simulink model "Approximation"  (R2024a)
settings: Solver=VariableStepAuto  StartTime=0.0  StopTime=15  RelTol=1e-3
values from neighbouring files (symbols this model uses):
  K = K(:,:,VeloIndexK)    [loadSystem.m]
  relOutput = 1:1:length(K.InputName)    [loadSystem.m]
  sysOL = sysOL(relOutput,:,VeloIndexSys)    [loadSystem.m]
settings Model: Creator=sp-ma  LastModifiedBy=sp-ma

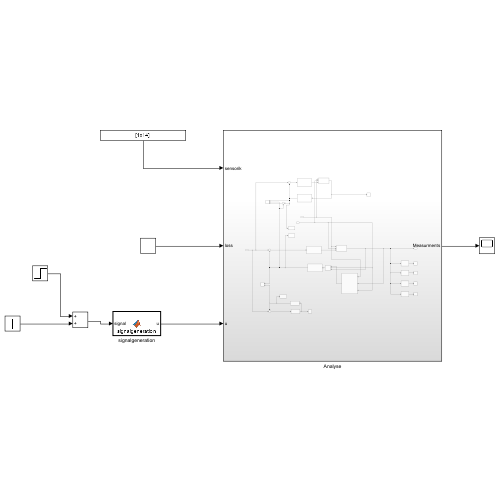
[thumbnail: Simulink's stored preview of the top-level diagram]
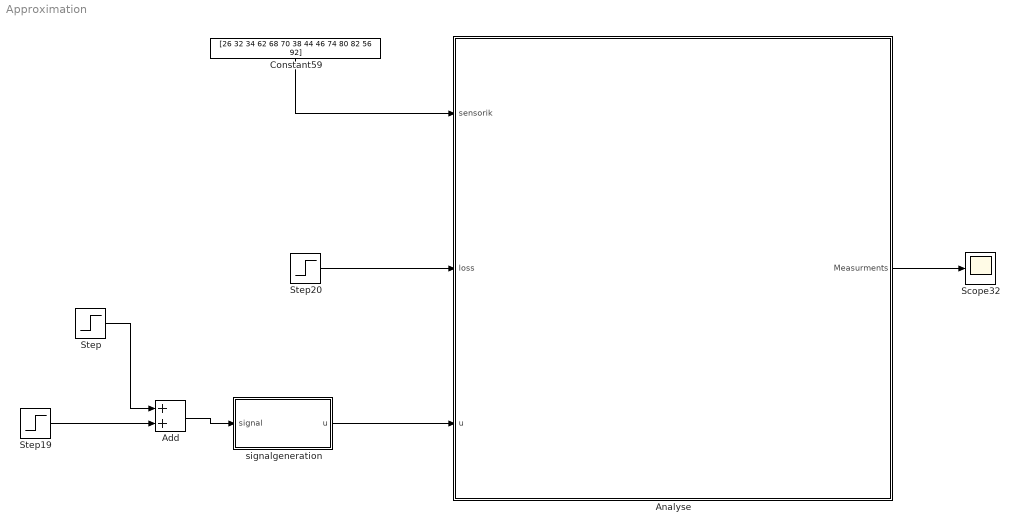
== system Approximation ==
  Add : Sum
  Analyse : Subsystem
  Constant59 : Constant  Value=[26 32 34 62 68 70 38 44 46 74 80 82 56 92]  VectorParams1D=off
  Scope32 : Scope
  Step : Step  Time=0.5  After=0  SampleTime=0
  Step19 : Step  Before=0.1  After=0.1  SampleTime=0
  Step20 : Step  Time=0.5  Before=1  SampleTime=0
  signalgeneration : MATLAB Function  TreatAsAtomicUnit=on
  wires:
  Constant59/1 -> Analyse/1(sensorik)
  Step20/1 -> Analyse/2(loss)
  signalgeneration/1(u) -> Analyse/3(u)
  Analyse/1(Measurments) -> Scope32/1
  Step19/1 -> Add/2
  Step/1 -> Add/1
  Add/1 -> signalgeneration/1(signal)

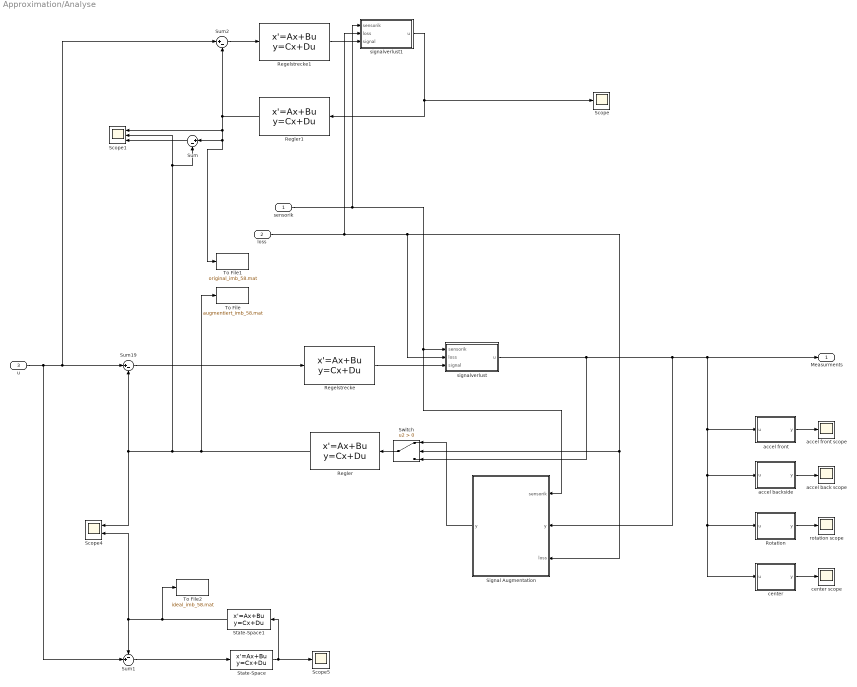
== system Approximation/Analyse ==
  sensorik : Inport
  loss : Inport  Port=2
  u : Inport  Port=3
  Regelstrecke : StateSpace  A=sysOL.A  B=sysOL.B  C=sysOL.C  D=sysOL.D  InitialCondition=0
  Regelstrecke1 : StateSpace  A=sysOL.A  B=sysOL.B  C=sysOL.C  D=sysOL.D  InitialCondition=0
  Regler : StateSpace  A=K.A  B=K.B  C=K.C  D=K.D  InitialCondition=0
  Regler1 : StateSpace  A=K.A  B=K.B  C=K.C  D=K.D  InitialCondition=0
  Rotation : MATLAB Function  TreatAsAtomicUnit=on
  Scope : Scope
  Scope1 : Scope  NumInputPorts=3
  Scope4 : Scope  NumInputPorts=2
  Scope5 : Scope
  Signal Augmentation : Subsystem
  State-Space : StateSpace  A=sysOL.A  B=sysOL.B  C=sysOL.C(relOutput,:)  D=sysOL.D(relOutput,:)  InitialCondition=0
  State-Space1 : StateSpace  A=K.A  B=K.B  C=K.C  D=K.D  InitialCondition=0
  Sum : Sum  Inputs=|+-
  Sum1 : Sum  Inputs=-+|
  Sum19 : Sum  Inputs=|+-
  Sum2 : Sum  Inputs=|+-
  Switch : Switch  Criteria=u2 > Threshold  SaturateOnIntegerOverflow=off  InputSameDT=off
  To File : ToFile  Filename=augmentiert_imb_58.mat
  To File1 : ToFile  Filename=original_imb_58.mat
  To File2 : ToFile  Filename=ideal_imb_58.mat
  accel back scope : Scope
  accel backside : MATLAB Function  TreatAsAtomicUnit=on
  accel front : MATLAB Function  TreatAsAtomicUnit=on
  accel front scope : Scope
  center : MATLAB Function  TreatAsAtomicUnit=on
  center scope : Scope
  rotation scope : Scope
  signalverlust : MATLAB Function  TreatAsAtomicUnit=on
  signalverlust1 : MATLAB Function  TreatAsAtomicUnit=on
  Measurments : Outport
  wires:
  sensorik/1 -> signalverlust1/1(sensorik), signalverlust/1(sensorik), Signal Augmentation/1(sensorik)
  u/1 -> Sum1/2, Sum2/1, Sum19/1
  Regelstrecke/1 -> signalverlust/3(signal)
  Regler/1 -> To File/1, Sum/2, Scope1/2, Sum19/2, Scope4/1
  Switch/1 -> Regler/1
  Rotation/1(y) -> rotation scope/1
  accel backside/1(y) -> accel back scope/1
  accel front/1(y) -> accel front scope/1
  signalverlust/1(u) -> accel front/1(u), accel backside/1(u), center/1(u), Rotation/1(u), Measurments/1, Signal Augmentation/2("y "), Switch/3
  loss/1 -> signalverlust1/2(loss), Signal Augmentation/3(loss), Switch/2, signalverlust/2(loss)
  Signal Augmentation/1(y) -> Switch/1
  State-Space1/1 -> To File2/1, Sum1/1, Scope4/2
  Sum1/1 -> State-Space/1
  State-Space/1 -> Scope5/1, State-Space1/1
  center/1(y) -> center scope/1
  Sum19/1 -> Regelstrecke/1
  Regelstrecke1/1 -> signalverlust1/3(signal)
  signalverlust1/1(u) -> Scope/1, Regler1/1
  Sum2/1 -> Regelstrecke1/1
  Regler1/1 -> To File1/1, Sum/1, Scope1/1, Sum2/2
  Sum/1 -> Scope1/3

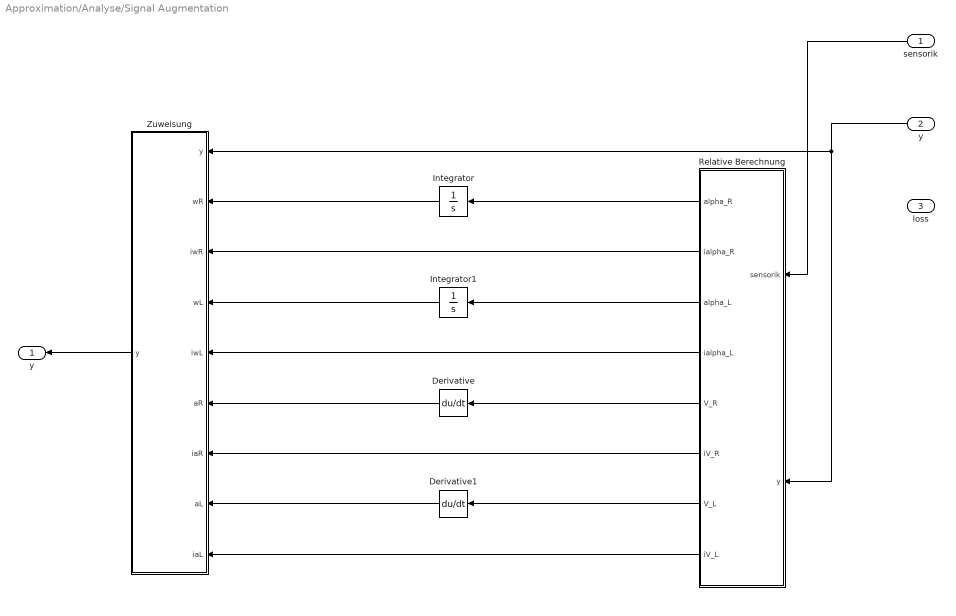
== system Approximation/Analyse/Signal Augmentation ==
  sensorik : Inport
  "y " : Inport  Port=2
  loss : Inport  Port=3
  Derivative : Derivative
  Derivative1 : Derivative
  Integrator : Integrator
  Integrator1 : Integrator
  Relative Berechnung : MATLAB Function  TreatAsAtomicUnit=on
  Zuweisung : MATLAB Function  TreatAsAtomicUnit=on
  y : Outport
  wires:
  Relative Berechnung/5(V_R) -> Derivative/1
  Relative Berechnung/6(iV_R) -> Zuweisung/7(iaR)
  Relative Berechnung/1(alpha_R) -> Integrator/1
  sensorik/1 -> Relative Berechnung/1(sensorik)
  Zuweisung/1(y) -> y/1
  Relative Berechnung/2(ialpha_R) -> Zuweisung/3(iwR)
  Relative Berechnung/8(iV_L) -> Zuweisung/9(iaL)
  Derivative1/1 -> Zuweisung/8(aL)
  Integrator/1 -> Zuweisung/2(wR)
  Relative Berechnung/4(ialpha_L) -> Zuweisung/5(iwL)
  Relative Berechnung/3(alpha_L) -> Integrator1/1
  Relative Berechnung/7(V_L) -> Derivative1/1
  "y "/1 -> Relative Berechnung/2(y), Zuweisung/1("y ")
  Derivative/1 -> Zuweisung/6(aR)
  Integrator1/1 -> Zuweisung/4(wL)

== matlab function Approximation/Analyse/center ==
  data: u input; y output
function y = fcn(u)
rot = [7 12];
y = u(rot);

== matlab function Approximation/Analyse/signalverlust1 ==
  data: sensorik input; loss input; u output; signal input
function u = signalverlust(sensorik,loss,signal)

if(loss~=0)
    signal(sensorik)=0;
end
u=signal;

== matlab function Approximation/signalgeneration ==
  data: u output; signal input
function u = signalgeneration(signal)
% t =0:10;
command = zeros(19,1);
% ilaileron = 13;
% iraileron = 14;
% command([15:19])=sin(t);
% % command([iraileron])=-1;

command([15 16]) = signal;
command([17 18]) = signal;
u=command;

== matlab function Approximation/Analyse/signalverlust ==
  data: sensorik input; loss input; u output; signal input
function u = signalverlust(sensorik,loss,signal)

if(loss~=0)
    signal(sensorik)=0;
end
u=signal;

== matlab function Approximation/Analyse/accel front ==
  data: u input; y output
function y = fcn(u)
fw = [26 38 50 62 74 86];
y = u(fw);

== matlab function Approximation/Analyse/accel backside ==
  data: u input; y output
function y = fcn(u)
bw = [32 44 56 68 80 92];
y = u(bw);

== matlab function Approximation/Analyse/Rotation ==
  data: u input; y output
function y = fcn(u)
rot = [34 46 58 70 82 94];
y = u(rot);

== matlab function Approximation/Analyse/Signal Augmentation/Relative Berechnung ==
  data: sensorik input; alpha_R output; ialpha_R output; alpha_L output; ialpha_L output; y input; V_R output; iV_R output; V_L output; iV_L output
function [alpha_R,ialpha_R,alpha_L,ialpha_L,V_R,iV_R,V_L,iV_L] = fcn(sensorik,y)

%Indexe der Sensoren der Flügelquerschnitte links und rechts fw=forward;
%bw = backward; rot = rotation
    Rfw =  [62 74 86];
    Rbw =  [68 80 92];
    Rrot = [70 82 94];
    R = [Rfw;Rbw;Rrot];
    R_lookup=R;
    Lfw =  [26 38 50];
    Lbw =  [32 44 56];
    Lrot = [34 46 58];
    L = [Lfw;Lbw;Lrot];
    L_lookup=L;
    
%Coordinaten der Sensoren
    Rcoord=[415, 1061;...
            602, 1061;...
            789, 2121;...
            933, 2121;...
            1164, 3183;...
            1260, 3182];
    Lcoord=[415, -1061;...
            602, -1061;...
            789, -2123;...
            933, -2120;...
            1164, -3184;...
            1260, -3183];

%initierung der Vektoren für die Codegenerierung
    alpha_R=zeros(1,3);
    ialpha_R=zeros(1,3);
    alpha_L=zeros(1,3);
    ialpha_L=zeros(1,3);
    V_R=zeros(1,3);
    iV_R=zeros(1,3);
    V_L=zeros(1,3);
    iV_L=zeros(1,3);
    xR=[Rcoord(2,1)-Rcoord(1,1),Rcoord(4,1)-Rcoord(3,1),Rcoord(6,1)-Rcoord(5,1)]/10^3;
    xL=[Lcoord(2,1)-Lcoord(1,1),Lcoord(4,1)-Lcoord(3,1),Lcoord(6,1)-Lcoord(5,1)]/10^3;
    x=xR;
    
    %% Überprüfen ob mehr als ein Element in einer Sensorreihe fehlerhaft ist
    for l=1:length(sensorik)
        R(R==sensorik(l))=0;
        L(L==sensorik(l))=0;
    end
    % disp(R)
    % disp(L)
    
%nachschauen welche Reihen ersetzt werden können. Wenn noch 2 Sensoren
%im Flügelquerschnitt funktionieren kann das Signal approximiert werden
    numberR=3*ones(1,3);
    numberL=3*ones(1,3);
    for i=1:3
        numberR(i)=nnz(R(:,i));
        numberL(i)=nnz(L(:,i));
    end
    % disp(numberR)
    % disp(numberL)
    
    right=find(numberR==2);
    left=find(numberL==2);
    % disp(right)
    % disp(left)
    
%Suche nach zu ersetzendem Signal und berechnen der direkt berechenbaren
%Größen. Werden ausgegeben und nachträglich je nach Sensor differenziert
%oder integriert.
    for l=1:length(right)
        row=find(R(:,right(l))==0);
        if row <=2
            V_R(l)=(y(R(3,right(l))))*xR(right(l));
            iV_R(l)=R_lookup(row,right(l));
        elseif row==3
            alpha_R(l)=(y(R(2,right(l)))-y(R(1,right(l))))/xR(i);
            ialpha_R(l)=R_lookup(row,right(l));
        end
    end
    for l=1:length(left)
        row=find(L(:,left(l))==0);
        if find(L(:,left(l))==0)<=2
            V_L(l)=(y(L(3,left(l))))*xL(left(l));
            iV_L(l)=L_lookup(row,left(l));
        elseif find(L(:,left(l))==0)==3
            alpha_L(l)=((y(L(2,left(l))))-(y(L(1,left(l)))))/xL(i);
            ialpha_L(l)=L_lookup(row,left(l));
        end
    end
end

== matlab function Approximation/Analyse/Signal Augmentation/Zuweisung ==
  data: y input; y output; wR input; iwR input; wL input; iwL input; aR input; iaR input; aL input; iaL input
function y = zuweisung(y,wR,iwR,wL,iwL,aR,iaR,aL,iaL)
%Indizes der Sensoren sammeln
    Rfw =  [62 74 86];
    Rbw =  [68 80 92];
    Rrot = [70 82 94];
    R=[Rfw;Rbw;Rrot];
    
    Lfw =  [26 38 50];
    Lbw =  [32 44 56];
    Lrot = [34 46 58];
    L=[Lfw;Lbw;Lrot];
    
% Wenn ein Eintrag im Vektor vorhanden ist, bedeutet dies dass dieser Sensor
% ersetzt werden muss
% Danach wird überprüft ob es sich um einen Beschleunigungs oder einen
% Rotationssensor handelt und es wird eine entsprechende Anpassung des
% Signals durchgeführt
% Rotation: das integrierte Signal wird eingefügt
% Beschleunigung: Differentieres Signal wird mit dem funktionierenden
% Beschleunigungssignal addiert.

% iaR = index der Beschleunigung von Sensor am rechten Flügel
% iwR = index der Rotation von Sensor am rechten Flügel
    if ~isempty(iaR)
        for l=1:length(iaR)
            [r,c]=find(R==iaR(l));
            if r==1
                y(R(r,c))=aR(l)+y(R(r+1,c));
            elseif r==2
                y(R(r,c))=aR(l)+y(R(r+1,c));
            end
        end
    end
    if ~isempty(iaL)
        for l=1:length(iaL)
            [r,c]=find(L==iaL(l));
            if r==1
                y(L(r,c))=aL(l)+y(L(r+1,c));
            elseif r==2
                y(L(r,c))=aL(l)+y(L(r+1,c));
            end
        end
    end
    if ~isempty(iwR)
        for l=1:length(iwR)
            [r,c]=find(R==iwR(l));
            y(R(r,c))=wR(l);
        end
    end
    if ~isempty(iwL)
        for l=1:length(iwL)
            [r,c]=find(L==iwL(l));
            y(L(r,c))=wL(l);
        end
    end

end
